simulink model "Copy_of_UAV"  (R2018b)
settings: Solver=FixedStepAuto  StartTime=0  StopTime=300  MaxStep=0.01  RelTol=1e-4  EnableMultiTasking=on
values from neighbouring files (symbols this model uses):
  actuatorCentres = 0.0    [data.sldd]
  datcom1 : value not decoded    [data.sldd]
  deflectionLimits = -10.0    [data.sldd]
  loggingSampleTime = 1.0    [data.sldd]
  sensorSampleTime = 0.02    [data.sldd]
  vehicle = 1.5    [data.sldd]
undefined symbols (not defined in the file or in its folder): aeroCoeff, DiscIntNeverNeededParam, Discrete, HDBK, MIL, Time
libraries: simulink x24, arduinolib x8, ctrlSharedLib x8, aerolibasang x5, aerolibactuator x4, aerolibadyn x3, aerolibconvert2 x2, aerolibatmos2 x2, aerolibnav x2, shared6dof x1, aerolibwind2 x1, simulink_extras x1
(part 1 of 3)
settings Model: DataDictionary=data.sldd  VariantConfigurationObject=Variants  SimulationMode=accelerator  SnapshotBufferSize=2  SnapshotInterval=1  PacingRate=10  ExtModeTrigDuration=2  Creator=Aliak  LastModifiedBy=Aliak
settings SolverCC: SolverResetMethod=Robust  MinimalZcImpactIntegration=on
settings OptimizationCC: DefaultParameterBehavior=Inlined  UseDivisionForNetSlopeComputation=on  UseFloatMulNetSlope=on  DefaultUnderspecifiedDataType=single  UseSpecifiedMinMax=on  InlineInvariantSignals=on  EnhancedBackFolding=on  BooleansAsBitfields=on  PassReuseOutputArgsAs=Individual arguments  StateBitsets=on  DataBitsets=on  ZeroExternalMemoryAtStartup=off  ZeroInternalMemoryAtStartup=off  NoFixptDivByZeroProtection=on  EfficientFloat2IntCast=on  LifeSpan=0.01  MaxStackSize=64  SimCompilerOptimization=on  OptimizeBlockOrder=speed  DifferentSizesBufferReuse=on
settings DebuggingCC: ConsistencyChecking=warning  ReadBeforeWriteMsg=DisableAll  WriteAfterWriteMsg=DisableAll  WriteAfterReadMsg=DisableAll  SolverPrmCheckMsg=warning  ParameterTunabilityLossMsg=error  UniqueDataStoreMsg=error  BusObjectLabelMismatch=error  StateNameClashWarn=warning  ForceCombineOutputUpdateInSim=on
settings HardwareCC: ProdBitPerInt=16  ProdBitPerPointer=16  ProdBitPerSizeT=16  ProdBitPerPtrDiffT=16  ProdLargestAtomicFloat=None  ProdWordSize=8  ProdLongLongMode=on  ProdHWDeviceType=Atmel->AVR
settings ModelReferenceCC: UpdateModelReferenceTargets=IfOutOfDate  EnableParallelModelReferenceBuilds=on  ModelReferenceMinAlgLoopOccurrences=on
settings SFSimCC: SimUserIncludeDirs="\"nativelibs/include\" \"nativelibs/src\" \"nativelibs/build\""  SFSimEcho=off  MATLABDynamicMemAlloc=off
settings RTWCC: SystemTargetFile=ert.tlc  HardwareBoard=Arduino Uno  TemplateMakefile=ert_default_tmf  GenerateReport=on  RTWUseSimCustomCode=on  CustomInclude="\"nativelibs/include\" \"nativelibs/src\" \"nativelibs/build\""  Toolchain=Arduino AVR  BuildConfiguration=Faster Runs  IncludeHyperlinkInReport=on  LaunchReport=on  PortableWordSizes=on  CreateSILPILBlock=PIL  GenerateTraceInfo=on  GenerateTraceReport=on  GenerateTraceReportSl=on  GenerateTraceReportSf=on  GenerateTraceReportEml=on  GenerateCodeMetricsReport=on
settings CodeAppCC: ForceParamTrailComments=on  IgnoreCustomStorageClasses=off  OperatorAnnotations=on  SimulinkDataObjDesc=on  SFDataObjDesc=on  CustomSymbolStrGlobalVar=rt$N$M  CustomSymbolStrType=$N$M  CustomSymbolStrFcn=$N$M$F  CustomSymbolStrMacro=$N$M  InsertBlockDesc=on
settings ERTTargetCC: TargetLangStandard=C99 (ISO)  UtilityFuncGeneration=Shared location  IncludeMdlTerminateFcn=off  CombineSignalStateStructs=on  SuppressErrorStatus=on  SupportNonFinite=off  SupportComplex=off  SupportVariableSizeSignals=on  CastingMode=Standards  ERTFilePackagingFormat=CompactWithDataFile

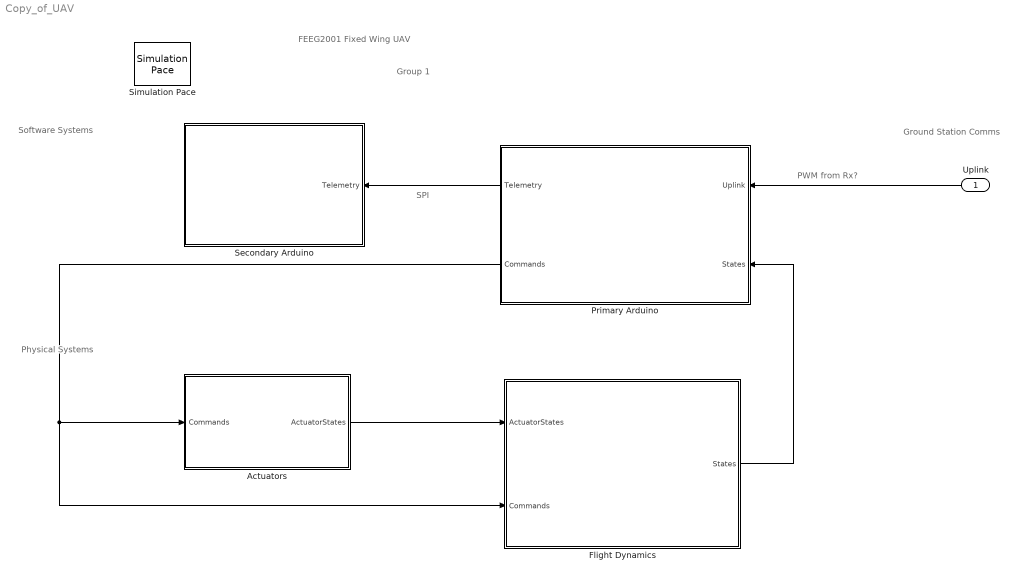
== system Copy_of_UAV ==
  note: PWM from Rx?
  note: SPI
  note: Group 1
  note: FEEG2001 Fixed Wing UAV
  note: Physical Systems
  note: Software Systems
  note: Ground Station Comms
  Uplink : Inport  OutDataTypeStr=Bus: Uplink
  Actuators : Subsystem  Variant=on
  Flight Dynamics : Subsystem
      mask Display: image('MQ-9-Reaper-armed-UAV.jpg');
  Primary Arduino : Subsystem
      mask Display: image('a000066_featured_1_.jpg');
  Secondary Arduino : Subsystem  VariantControl=Variant1
      mask Display: image('a000066_featured_1_.jpg');
  Simulation Pace : aerolibanimutils/Simulation Pace  SimulationPace=1  SleepMode=Auto  OutputPaceError=off  SampleTime=sensorSampleTime
  wires:
  Actuators/1(ActuatorStates) -> Flight Dynamics/1(ActuatorStates)
  Primary Arduino/2(Commands) -> Flight Dynamics/2(Commands), Actuators/1(Commands)
  Uplink/1 -> Primary Arduino/1(Uplink)
  Flight Dynamics/1(States) -> Primary Arduino/2(States)
  Primary Arduino/1(Telemetry) -> Secondary Arduino/1(Telemetry)

== system Copy_of_UAV/Actuators ==
  Commands : Inport
  Model Actuators : Subsystem  VariantControl=SimType == 0
  Real Actuators : Subsystem  VariantControl=SimType == 1
  ActuatorStates : Outport

== system Copy_of_UAV/Flight Dynamics ==
  ActuatorStates : Inport
  Commands : Inport  Port=2  OutDataTypeStr=Bus: Commands
  6DOF EOM : Subsystem  VariantControl=eom3DOF
  Bus Selector : BusSelector  OutputSignals=Throttle
  Coeff Model : Subsystem  Commented=on  VariantControl=AeroModel==2
  DATCOM Model : Subsystem  VariantControl=AeroModel==1
  Environment : Subsystem
  Propulsion : Subsystem
      settings: RTWSystemCode=Inline
  Sum1 : Sum  Inputs=|++  SaturateOnIntegerOverflow=on  InputSameDT=on  OutDataTypeStr=Inherit: Same as first input
  Sum2 : Sum  Inputs=|++  SaturateOnIntegerOverflow=on  InputSameDT=on  OutDataTypeStr=Inherit: Same as first input
  Visualization : Subsystem
  States : Outport
  wires:
  Commands/1 -> Bus Selector/1
  Sum2/1 -> 6DOF EOM/2(Forces)
  Propulsion/1(F) -> Sum2/2
  Propulsion/2(M) -> Sum1/2
  Sum1/1 -> 6DOF EOM/3(Moments)
  Bus Selector/1 -> Propulsion/1(cmd)  "<Throttle>"
  ActuatorStates/1 -> DATCOM Model/3(ActuatorStates)
  DATCOM Model/1(F) -> Sum2/1
  DATCOM Model/2(M) -> Sum1/1
  Environment/1(Env) -> 6DOF EOM/1(Env), DATCOM Model/1(Env)
  6DOF EOM/1(DCMbe) -> Environment/2(DCMbe)
  6DOF EOM/2(States) -> Environment/1(States), Visualization/1(States), DATCOM Model/2(States), States/1

== system Copy_of_UAV/Primary Arduino ==
  Uplink : Inport
  States : Inport  Port=2
  Communications : Subsystem
  Flight Control : Subsystem  VariantControlMode=Label  Variant=on  VariantControl=Variant1  LabelModeActiveChoice=SimType==0
  Rate Transition : RateTransition  OutPortSampleTime=loggingSampleTime
  Sensors : Subsystem  VariantControl=Variant1
  Telemetry and Errors : Subsystem  VariantControlMode=Label  Variant=on  VariantControl=Variant1  LabelModeActiveChoice=SecArd == 0
  Telemetry : Outport
  Commands : Outport  Port=2
  wires:
  Uplink/1 -> Communications/1(Uplink)
  Telemetry and Errors/1(" Telemetry") -> Telemetry/1
  States/1 -> Sensors/1(States)
  Sensors/1(Sensors) -> Rate Transition/1, Flight Control/2("Sensors ")
  Communications/1(Demands) -> Flight Control/1("Demands ")
  Flight Control/1(" Commands") -> Commands/1
  Rate Transition/1 -> Telemetry and Errors/1("Sensors ")

== system Copy_of_UAV/Secondary Arduino ==
  Telemetry : Inport
  Telemetry Logging : Subsystem  VariantControlMode=Label  Variant=on  VariantControl=Variant1  LabelModeActiveChoice=SecArd==0
  wires:
  Telemetry/1 -> Telemetry Logging/1("Telemetry ")

== system Copy_of_UAV/Actuators/Model Actuators ==
  Commands : Inport
  Bus Creator : BusCreator  Inputs=4  OutDataTypeStr=Bus: ActuatorStates
  Bus Selector : BusSelector  OutputSignals=Aileron,Elevator,Rudder,Flap
  Cast To Double{,1..3} (4 alike) : DataTypeConversion  OutDataTypeStr=double
  Linear Second-Order Actuator{,1..3} (4 alike) : aerolibactuator/Linear Second-Order Actuator  wn_fin=1  z_fin=0.3  fin_act_0=0  fin_act_vel=0
      settings: SourceProductName=Aerospace Blockset  SourceProductBaseCode=AE
  Saturation : Saturate  UpperLimit=deflectionLimits.aileron.max  LowerLimit=deflectionLimits.aileron.min
  Saturation1 : Saturate  UpperLimit=deflectionLimits.elevator.max  LowerLimit=deflectionLimits.elevator.min
  Saturation2 : Saturate  UpperLimit=deflectionLimits.rudder.max  LowerLimit=deflectionLimits.rudder.min
  Saturation3 : Saturate  UpperLimit=deflectionLimits.flap.max  LowerLimit=deflectionLimits.flap.min
  ActuatorStates : Outport
  wires:
  Bus Selector/3 -> Cast To Double2/1  "<Rudder>"
  Bus Selector/4 -> Cast To Double3/1  "<Flap>"
  Bus Selector/1 -> Cast To Double/1  "<Aileron>"
  Bus Selector/2 -> Cast To Double1/1  "<Elevator>"
  Saturation/1 -> Linear Second-Order Actuator/1
  Saturation1/1 -> Linear Second-Order Actuator1/1
  Saturation2/1 -> Linear Second-Order Actuator2/1
  Saturation3/1 -> Linear Second-Order Actuator3/1
  Linear Second-Order Actuator1/1 -> Bus Creator/2  "Elevator"
  Linear Second-Order Actuator/1 -> Bus Creator/1  "Aileron"
  Linear Second-Order Actuator2/1 -> Bus Creator/3  "Rudder"
  Linear Second-Order Actuator3/1 -> Bus Creator/4  "Flap"
  Bus Creator/1 -> ActuatorStates/1
  Commands/1 -> Bus Selector/1
  Cast To Double/1 -> Saturation/1
  Cast To Double1/1 -> Saturation1/1
  Cast To Double2/1 -> Saturation2/1
  Cast To Double3/1 -> Saturation3/1

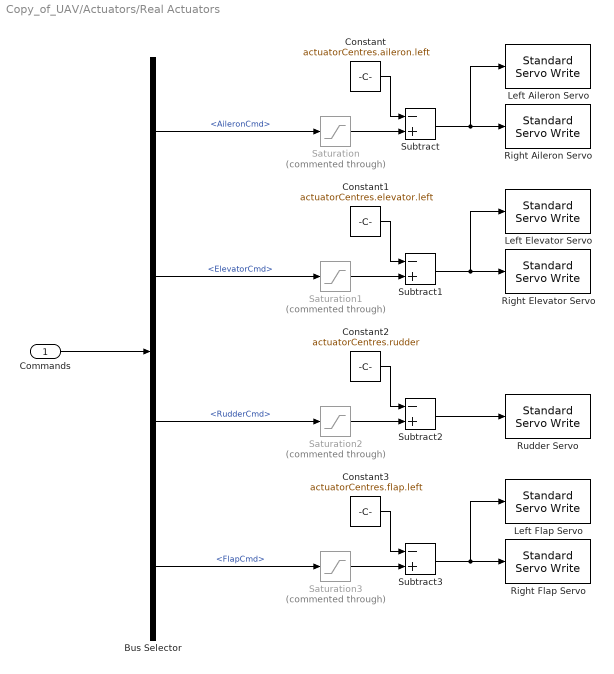
== system Copy_of_UAV/Actuators/Real Actuators ==
  Commands : Inport
  Bus Selector : BusSelector  OutputSignals=AileronCmd,ElevatorCmd,RudderCmd,FlapCmd
  Constant : Constant  Value=actuatorCentres.aileron.left
  Constant1 : Constant  Value=actuatorCentres.elevator.left
  Constant2 : Constant  Value=actuatorCentres.rudder
  Constant3 : Constant  Value=actuatorCentres.flap.left
  Left Aileron Servo : arduinolib/Standard Servo Write  pinNumber=servoPins.aileron.left  ServoIndex=0  blockPlatform=ARDUINO
      settings: SourceProductName=Simulink Support Package for Arduino Hardware
  Left Elevator Servo : arduinolib/Standard Servo Write  pinNumber=servoPins.elevator.left  ServoIndex=0  blockPlatform=ARDUINO
      settings: SourceProductName=Simulink Support Package for Arduino Hardware
  Left Flap Servo : arduinolib/Standard Servo Write  pinNumber=servoPins.flap.left  ServoIndex=0  blockPlatform=ARDUINO
      settings: SourceProductName=Simulink Support Package for Arduino Hardware
  Right Aileron Servo : arduinolib/Standard Servo Write  pinNumber=servoPins.aileron.right  ServoIndex=0  blockPlatform=ARDUINO
      settings: SourceProductName=Simulink Support Package for Arduino Hardware
  Right Elevator Servo : arduinolib/Standard Servo Write  pinNumber=servoPins.elevator.right  ServoIndex=0  blockPlatform=ARDUINO
      settings: SourceProductName=Simulink Support Package for Arduino Hardware
  Right Flap Servo : arduinolib/Standard Servo Write  pinNumber=servoPins.flap.right  ServoIndex=0  blockPlatform=ARDUINO
      settings: SourceProductName=Simulink Support Package for Arduino Hardware
  Rudder Servo : arduinolib/Standard Servo Write  pinNumber=servoPins.rudder  ServoIndex=0  blockPlatform=ARDUINO
      settings: SourceProductName=Simulink Support Package for Arduino Hardware
  Saturation : Saturate  Commented=through  UpperLimit=deflectionLimits.aileron.max  LowerLimit=deflectionLimits.aileron.min
  Saturation1 : Saturate  Commented=through  UpperLimit=deflectionLimits.elevator.max  LowerLimit=deflectionLimits.elevator.min
  Saturation2 : Saturate  Commented=through  UpperLimit=deflectionLimits.rudder.max  LowerLimit=deflectionLimits.rudder.min
  Saturation3 : Saturate  Commented=through  UpperLimit=deflectionLimits.flap.max  LowerLimit=deflectionLimits.flap.min
  Subtract{,1..3} (4 alike) : Sum  Inputs=-+
  wires:
  Saturation/1 -> Subtract/2
  Bus Selector/3 -> Saturation2/1  "<RudderCmd>"
  Commands/1 -> Bus Selector/1
  Bus Selector/4 -> Saturation3/1  "<FlapCmd>"
  Subtract3/1 -> Right Flap Servo/1, Left Flap Servo/1
  Bus Selector/1 -> Saturation/1  "<AileronCmd>"
  Constant2/1 -> Subtract2/1
  Subtract2/1 -> Rudder Servo/1
  Saturation3/1 -> Subtract3/2
  Saturation2/1 -> Subtract2/2
  Saturation1/1 -> Subtract1/2
  Bus Selector/2 -> Saturation1/1  "<ElevatorCmd>"
  Subtract/1 -> Right Aileron Servo/1, Left Aileron Servo/1
  Subtract1/1 -> Right Elevator Servo/1, Left Elevator Servo/1
  Constant/1 -> Subtract/1
  Constant1/1 -> Subtract1/1
  Constant3/1 -> Subtract3/1

== system Copy_of_UAV/Flight Dynamics/6DOF EOM ==
  Bus Element In : Inport  PortName=Env  Element=g
  Forces : Inport  Port=2
  Moments : Inport  Port=3
  6DOF (Euler Angles) : shared6dof/6DOF (Euler Angles)  units=Metric (MKS)  mtype=Fixed  rep=Euler Angles  xme_0=initConditions.x0  Vm_0=initConditions.v0  eul_0=initConditions.euler0  pm_0=initConditions.w0  mass_0=vehicle.mass  mass_e=0.5  mass_f=2.0  inertia=vehicle.inertia  inertia_e=eye(3)  inertia_f=2*eye(3)  k_quat=1.0  vre_flag=on  abi_flag=on  aMode=0  xme_statename=''  Vm_statename=''  eul_statename=''  quat_statename=''  pm_statename=''  mass_statename=''
      settings: SourceProductBaseCode=AE
  Gain : Gain  Gain=vehicle.mass
  Product : Product  Multiplication=Matrix(*)
  Sum2 : Sum  Inputs=++|  SaturateOnIntegerOverflow=on  InputSameDT=on  OutDataTypeStr=Inherit: Same as first input
  Terminator1 : Terminator
  Terminator2 : Terminator
  DCMbe : Outport
  Bus Element Out : Outport  Port=2  PortName=States  Element=phi_theta_psi
  Bus Element Out1 : Outport  Port=2  PortName=States  Element=pqr
  Bus Element Out2 : Outport  Port=2  PortName=States  Element=omega_dot
  Bus Element Out15 : Outport  Port=2  PortName=States  Element=X_e
  Bus Element Out16 : Outport  Port=2  PortName=States  Element=V_b
  Bus Element Out17 : Outport  Port=2  PortName=States  Element=A_be
  wires:
  6DOF (Euler Angles)/4 -> DCMbe/1, Product/1
  6DOF (Euler Angles)/1 -> Terminator2/1
  Bus Element In/1 -> Gain/1
  6DOF (Euler Angles)/9 -> Bus Element Out17/1
  6DOF (Euler Angles)/7 -> Bus Element Out2/1
  6DOF (Euler Angles)/6 -> Bus Element Out1/1
  6DOF (Euler Angles)/5 -> Bus Element Out16/1
  6DOF (Euler Angles)/3 -> Bus Element Out/1
  6DOF (Euler Angles)/2 -> Bus Element Out15/1
  Gain/1 -> Product/2
  Sum2/1 -> 6DOF (Euler Angles)/1
  Product/1 -> Sum2/1
  6DOF (Euler Angles)/8 -> Terminator1/1
  Moments/1 -> 6DOF (Euler Angles)/2
  Forces/1 -> Sum2/2

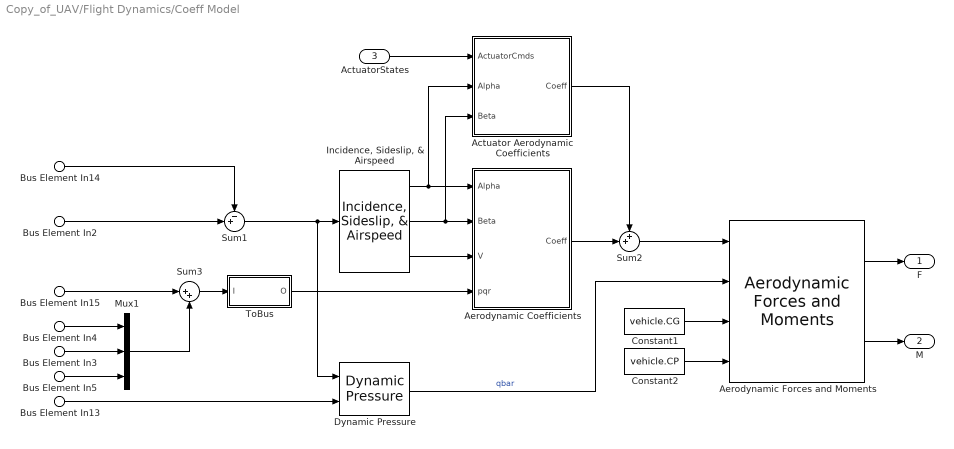
== system Copy_of_UAV/Flight Dynamics/Coeff Model ==
  Bus Element In13 : Inport  PortName=Env  Element=AirDensity
  Bus Element In14 : Inport  PortName=Env  Element=WindVelocity
  Bus Element In15 : Inport  PortName=Env  Element=WindAngularRates
  Bus Element In3 : Inport  Port=2  PortName=States  Element=q
  Bus Element In4 : Inport  Port=2  PortName=States  Element=p
  Bus Element In5 : Inport  Port=2  PortName=States  Element=r
  Bus Element In2 : Inport  Port=2  PortName=States  Element=V_b
  ActuatorStates : Inport  Port=3  OutDataTypeStr=Bus: ActuatorStates
  Actuator Aerodynamic Coefficients : Subsystem
  Aerodynamic Coefficients : Subsystem
  Aerodynamic Forces and Moments : aerolibadyn/Aerodynamic Forces and Moments   inputAxes=Body  outputForceAxes=Body  outputMomentAxes=Body  S=vehicle.wingarea  b=vehicle.wingspan  cbar=vehicle.aclength
      settings: SourceProductName=Aerospace Blockset
  Constant1 : Constant  Value=vehicle.CG
  Constant2 : Constant  Value=vehicle.CP
  Dynamic Pressure : aerolibasang/Dynamic Pressure
  "Incidence, Sideslip, & Airspeed" : aerolibasang/Incidence, Sideslip, & Airspeed
      settings: SourceProductName=Aerospace Blockset
  Mux1 : Mux  Inputs=3
  Sum1 : Sum  Inputs=-+|  SaturateOnIntegerOverflow=on  InputSameDT=on  OutDataTypeStr=Inherit: Same as first input
  Sum2 : Sum  Inputs=++|
  Sum3 : Sum  Inputs=|++  SaturateOnIntegerOverflow=on  InputSameDT=on  OutDataTypeStr=Inherit: Same as first input
  ToBus : Subsystem
  F : Outport  Unit=N
  M : Outport  Port=2  Unit=N*m
  wires:
  ActuatorStates/1 -> Actuator Aerodynamic Coefficients/1(ActuatorCmds)
  Bus Element In14/1 -> Sum1/1
  Bus Element In2/1 -> Sum1/2
  Mux1/1 -> Sum3/2
  Bus Element In15/1 -> Sum3/1
  Bus Element In5/1 -> Mux1/3
  Bus Element In3/1 -> Mux1/2
  Bus Element In4/1 -> Mux1/1
  Actuator Aerodynamic Coefficients/1(Coeff) -> Sum2/1
  Aerodynamic Coefficients/1(Coeff) -> Sum2/2
  ToBus/1(O) -> Aerodynamic Coefficients/4(pqr)
  Sum1/1 -> Dynamic Pressure/1, "Incidence, Sideslip, & Airspeed"/1
  Dynamic Pressure/1 -> Aerodynamic Forces and Moments/2  "qbar"
  Sum3/1 -> ToBus/1(I)
  Bus Element In13/1 -> Dynamic Pressure/2
  "Incidence, Sideslip, & Airspeed"/3 -> Aerodynamic Coefficients/3(V)
  "Incidence, Sideslip, & Airspeed"/2 -> Aerodynamic Coefficients/2(Beta), Actuator Aerodynamic Coefficients/3(Beta)
  Aerodynamic Forces and Moments/2 -> M/1
  Aerodynamic Forces and Moments/1 -> F/1
  Constant2/1 -> Aerodynamic Forces and Moments/4
  Constant1/1 -> Aerodynamic Forces and Moments/3
  Sum2/1 -> Aerodynamic Forces and Moments/1
  "Incidence, Sideslip, & Airspeed"/1 -> Actuator Aerodynamic Coefficients/2(Alpha), Aerodynamic Coefficients/1(Alpha)

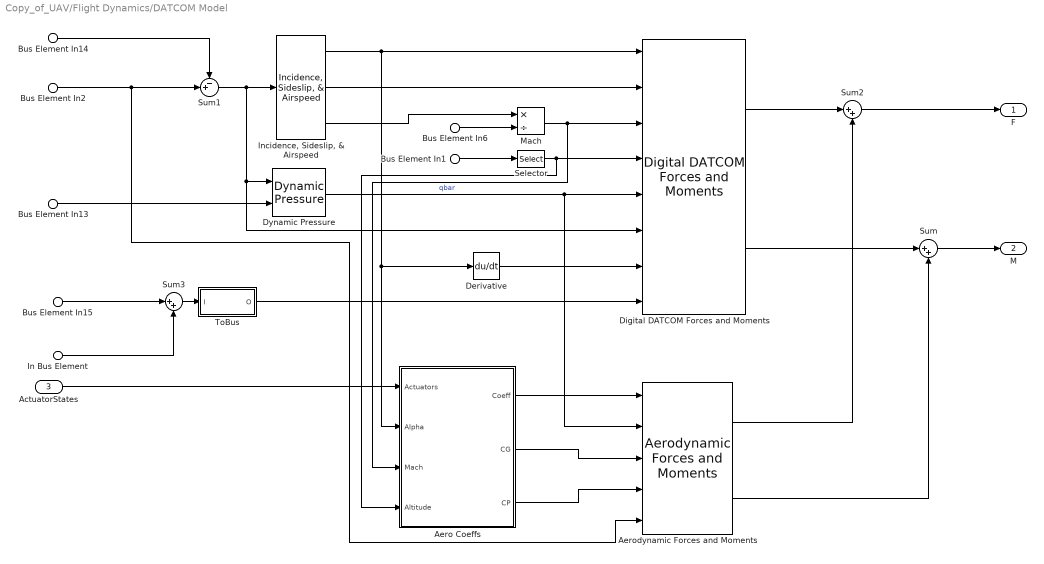
== system Copy_of_UAV/Flight Dynamics/DATCOM Model ==
  Bus Element In13 : Inport  PortName=Env  Element=AirDensity
  Bus Element In14 : Inport  PortName=Env  Element=WindVelocity
  Bus Element In15 : Inport  PortName=Env  Element=WindAngularRates
  Bus Element In6 : Inport  PortName=Env  Element=a
  Bus Element In2 : Inport  Port=2  PortName=States  Element=V_b
  Bus Element In1 : Inport  Port=2  PortName=States  Element=X_e
  In Bus Element : Inport  Port=2  PortName=States  Element=pqr
  ActuatorStates : Inport  Port=3  OutDataTypeStr=Bus: ActuatorStates
  Aero Coeffs : Subsystem
  "Aerodynamic Forces and Moments " : aerolibadyn/Aerodynamic Forces and Moments   inputAxes=Stability  outputForceAxes=Body  outputMomentAxes=Body  S=vehicle.wingarea  b=vehicle.wingspan  cbar=vehicle.cbar
      settings: SourceProductName=Aerospace Blockset
  Derivative : Derivative
  Digital DATCOM Forces and Moments : aerolibadyn/Digital DATCOM Forces and Moments  units=Metric (MKS)  dcase=datcom1{3}  fmode=Body  buildno=0  imethod=Linear  emethod=Linear  rmethod=Linear Extrapolation  action=Warning
      settings: SourceProductName=Aerospace Blockset  SourceProductBaseCode=AE
  Dynamic Pressure : aerolibasang/Dynamic Pressure
  "Incidence, Sideslip, & Airspeed" : aerolibasang/Incidence, Sideslip, & Airspeed
      settings: SourceProductName=Aerospace Blockset
  Mach : Product  Inputs=*/
  Selector : Selector  IndexMode=Zero-based  InputPortWidth=3  IndexOptions=Index vector (dialog)  Indices=[2]  OutputSizes=1
  Sum : Sum  Inputs=|++
  Sum1 : Sum  Inputs=-+|  SaturateOnIntegerOverflow=on  InputSameDT=on  OutDataTypeStr=Inherit: Same as first input
  Sum2 : Sum  Inputs=|++
  Sum3 : Sum  Inputs=|++  SaturateOnIntegerOverflow=on  InputSameDT=on  OutDataTypeStr=Inherit: Same as first input
  ToBus : Subsystem
  F : Outport  Unit=N
  M : Outport  Port=2  Unit=N*m
  wires:
  Bus Element In14/1 -> Sum1/1
  Bus Element In2/1 -> "Aerodynamic Forces and Moments "/5, Sum1/2
  In Bus Element/1 -> Sum3/2
  Bus Element In15/1 -> Sum3/1
  Sum1/1 -> "Incidence, Sideslip, & Airspeed"/1, Digital DATCOM Forces and Moments/6, Dynamic Pressure/1
  Sum3/1 -> ToBus/1(I)
  Bus Element In13/1 -> Dynamic Pressure/2
  "Incidence, Sideslip, & Airspeed"/3 -> Mach/1
  Digital DATCOM Forces and Moments/2 -> Sum/1
  Digital DATCOM Forces and Moments/1 -> Sum2/1
  Dynamic Pressure/1 -> "Aerodynamic Forces and Moments "/2, Digital DATCOM Forces and Moments/5  "qbar"
  Bus Element In1/1 -> Selector/1
  Selector/1 -> Aero Coeffs/4(Altitude), Digital DATCOM Forces and Moments/4
  Bus Element In6/1 -> Mach/2
  ActuatorStates/1 -> Aero Coeffs/1(Actuators)
  "Incidence, Sideslip, & Airspeed"/2 -> Digital DATCOM Forces and Moments/2
  "Incidence, Sideslip, & Airspeed"/1 -> Digital DATCOM Forces and Moments/1, Derivative/1, Aero Coeffs/2(Alpha)
  Aero Coeffs/1(Coeff) -> "Aerodynamic Forces and Moments "/1
  Aero Coeffs/2(CG) -> "Aerodynamic Forces and Moments "/3
  Aero Coeffs/3(CP) -> "Aerodynamic Forces and Moments "/4
  Sum/1 -> M/1
  "Aerodynamic Forces and Moments "/2 -> Sum/2
  Sum2/1 -> F/1
  "Aerodynamic Forces and Moments "/1 -> Sum2/2
  ToBus/1(O) -> Digital DATCOM Forces and Moments/8
  Derivative/1 -> Digital DATCOM Forces and Moments/7
  Mach/1 -> Digital DATCOM Forces and Moments/3, Aero Coeffs/3(Mach)

== system Copy_of_UAV/Flight Dynamics/Environment ==
  States : Inport
  DCMbe : Inport  Port=2
  Bus Creator : BusCreator  Inputs=5
  Bus Selector : BusSelector  OutputSignals=X_e,V_b
  Dryden Wind Turbulence Model (Discrete (-q +r)) : aerolibwind2/Dryden Wind Turbulence Model  (Continuous (+q -r))  units=Metric (MKS)  spec=MIL-HDBK-1797  model=Discrete Dryden (-q +r)  W20=1  Wdeg=250  TurbProb=10^-1  L_high=533.4  Wingspan=1.8  ts=sensorSampleTime  Seed=[23341 23342 23343 23344]  T_on=off
      settings: SourceProductName=Aerospace Blockset
  Lapse Rate Model : aerolibatmos2/ISA Atmosphere Model  custom=off  g=9.80665  gamma=1.4  R=287.0531  L=0.0065  h_trop=11000  h_strat=20000  rho0=1.225  P0=101325  T0=288.15  h0=0
      settings: SourceProductName=Aerospace Blockset
  Selector : Selector  IndexMode=Zero-based  InputPortWidth=3  IndexOptions=Index vector (dialog)  Indices=[0]  OutputSizes=1
  Selector1 : Selector  IndexMode=Zero-based  InputPortWidth=3  IndexOptions=Index vector (dialog)  Indices=[0]  OutputSizes=1
  Terminator : Terminator
  Terminator1 : Terminator
  g : Constant  Value=[0 0 9.80665]
  Env : Outport
  wires:
  States/1 -> Bus Selector/1
  Bus Creator/1 -> Env/1
  Selector/1 -> Dryden Wind Turbulence Model (Discrete (-q +r))/1, Lapse Rate Model/1
  Bus Selector/1 -> Selector/1  "<X_e>"
  Lapse Rate Model/4 -> Bus Creator/2  "AirDensity"
  Lapse Rate Model/2 -> Bus Creator/1  "a"
  g/1 -> Bus Creator/3  "g"
  DCMbe/1 -> Dryden Wind Turbulence Model (Discrete (-q +r))/3
  Bus Selector/2 -> Selector1/1  "<V_b>"
  Selector1/1 -> Dryden Wind Turbulence Model (Discrete (-q +r))/2
  Dryden Wind Turbulence Model (Discrete (-q +r))/1 -> Bus Creator/4  "WindVelocity"
  Dryden Wind Turbulence Model (Discrete (-q +r))/2 -> Bus Creator/5  "WindAngularRates"
  Lapse Rate Model/1 -> Terminator/1
  Lapse Rate Model/3 -> Terminator1/1

== system Copy_of_UAV/Flight Dynamics/Propulsion ==
  cmd : Inport  OutDataTypeStr=single
  Cast To Double : DataTypeConversion  OutDataTypeStr=double
  Mux : Mux  Inputs=[1 2]
  Product : Product
  ThrustX : Lookup_n-D  NumberOfTableDimensions=1  LookupTableObject=''  BreakpointsForDimension1=(1/6)*(3+([-3:3]))  IndexSearchMethod=Linear search  BeginIndexSearchUsingPreviousIndexResult=on  Table=vehicle.thrust*(1+tanh([-3:3]))  ExtrapMethod=Clip  InternalRulePriority=Speed
  ThrustYZ : Constant  Value=[0 0]'  SampleTime=-1
  Thrust_M1 : Constant  Value=[-0.1 0 0.01]  SampleTime=-1
  Vector Concatenate : Concatenate
  F : Outport  Unit=N
  M : Outport  Port=2  Unit=N*m
  wires:
  Thrust_M1/1 -> Product/2
  ThrustX/1 -> Mux/1, Vector Concatenate/2
  ThrustYZ/1 -> Vector Concatenate/1, Mux/2
  Mux/1 -> F/1
  cmd/1 -> Cast To Double/1
  Product/1 -> M/1
  Vector Concatenate/1 -> Product/1
  Cast To Double/1 -> ThrustX/1

== system Copy_of_UAV/Flight Dynamics/Visualization ==
  Bus Element In3 : Inport  PortName=States  Element=pqr
  Bus Element In9 : Inport  PortName=States  Element=X_e
  In Bus Element : Inport  PortName=States  Element=V_b
  In Bus Element1 : Inport  PortName=States  Element=phi_theta_psi
  "Incidence, Sideslip, & Airspeed" : aerolibasang/Incidence, Sideslip, & Airspeed
      settings: SourceProductName=Aerospace Blockset
  Mux5 : Mux  Inputs=2
  State Plots : Scope  NumInputPorts=4
  Terminator : Terminator
  wires:
  Bus Element In9/1 -> State Plots/4
  In Bus Element1/1 -> State Plots/2
  Mux5/1 -> State Plots/1
  "Incidence, Sideslip, & Airspeed"/2 -> Mux5/2  "beta"
  "Incidence, Sideslip, & Airspeed"/1 -> Mux5/1  "alpha"
  In Bus Element/1 -> "Incidence, Sideslip, & Airspeed"/1
  Bus Element In3/1 -> State Plots/3
  "Incidence, Sideslip, & Airspeed"/3 -> Terminator/1

== system Copy_of_UAV/Primary Arduino/Communications ==
  Uplink : Inport  OutDataTypeStr=Bus: Uplink
  Bus Creator : BusCreator  Inputs=5  OutDataTypeStr=Bus: Demands
      settings: InheritFromInputs=off
  Bus Selector : BusSelector  OutputSignals=AutoflightRefValues,Override,ControlOverride
  Bus Selector1 : BusSelector  OutputSignals=FlightMode,HoldAltitude,HoldHeading
  Demands : Outport  OutDataTypeStr=Bus: Demands
  wires:
  Uplink/1 -> Bus Selector/1
  Bus Selector/1 -> Bus Selector1/1  "<AutoflightRefValues>"
  Bus Selector1/1 -> Bus Creator/1  "<FlightMode>"
  Bus Selector1/2 -> Bus Creator/2  "<HoldAltitude>"
  Bus Selector1/3 -> Bus Creator/3  "<HoldHeading>"
  Bus Creator/1 -> Demands/1
  Bus Selector/3 -> Bus Creator/5  "<ControlOverride>"
  Bus Selector/2 -> Bus Creator/4  "<Override>"

== system Copy_of_UAV/Primary Arduino/Flight Control ==
  "Demands " : Inport
  "Sensors " : Inport  Port=2
  Model Flight Control : Subsystem  VariantControl=SimType==0
  Real Flight Control : Subsystem  VariantControl=SimType==1
  " Commands" : Outport

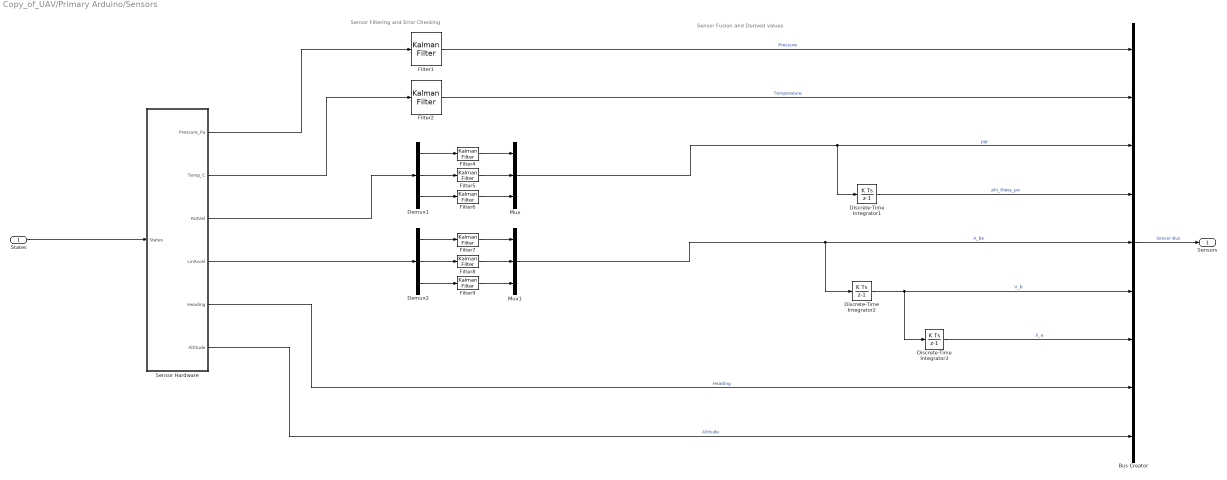
== system Copy_of_UAV/Primary Arduino/Sensors ==
  note: Sensor Fusion and Derived values
  note: Sensor Filtering and Error Checking
  States : Inport
  Bus Creator : BusCreator  Inputs=9  OutDataTypeStr=Bus: Sensors
  Demux1 : Demux  Outputs=3
  Demux2 : Demux  Outputs=3
  Discrete-Time Integrator1 : DiscreteIntegrator  SampleTime=sensorSampleTime  ICPrevOutput=DiscIntNeverNeededParam  ICPrevScaledInput=DiscIntNeverNeededParam
  Discrete-Time Integrator2 : DiscreteIntegrator  SampleTime=sensorSampleTime  ICPrevOutput=DiscIntNeverNeededParam  ICPrevScaledInput=DiscIntNeverNeededParam
  Discrete-Time Integrator3 : DiscreteIntegrator  SampleTime=sensorSampleTime  ICPrevOutput=DiscIntNeverNeededParam  ICPrevScaledInput=DiscIntNeverNeededParam
  Filter1 : ctrlSharedLib/Kalman Filter  TimeDomain=Discrete-Time  UseCurrentEstimator=on  ModelSource=Individual A, B, C, D matrices  ModelSourceVariable=ss(1,[],1,[],1)  A=0.95  B=1  C=1  D=0  NumberOfStates=1  NumberOfInputs=1  NumberOfOutputs=1  InitialEstimateSource=Dialog  X0=101325  P0=10  UseK=off  UseGH=off  NumberOfProcessNoiseInputs=1  G=1  TimeInvariantG=on  H=0  TimeInvariantH=on  Q=0.05  TimeInvariantQ=on  R=1  TimeInvariantR=on  N=0  TimeInvariantN=on  AddInputPort=off  AddEnablePort=off  OutputEstimatedY=off  OutputP=off  Ts=sensorSampleTime
      settings: SourceProductBaseCode=CT
  Filter2 : ctrlSharedLib/Kalman Filter  TimeDomain=Discrete-Time  UseCurrentEstimator=on  ModelSource=Individual A, B, C, D matrices  ModelSourceVariable=ss(1,[],1,[],1)  A=0.95  B=1  C=1  D=0  NumberOfStates=1  NumberOfInputs=1  NumberOfOutputs=1  InitialEstimateSource=Dialog  X0=15  P0=10  UseK=off  UseGH=off  NumberOfProcessNoiseInputs=1  G=1  TimeInvariantG=on  H=0  TimeInvariantH=on  Q=0.05  TimeInvariantQ=on  R=1  TimeInvariantR=on  N=0  TimeInvariantN=on  AddInputPort=off  AddEnablePort=off  OutputEstimatedY=off  OutputP=off  Ts=sensorSampleTime
      settings: SourceProductBaseCode=CT
  Filter4 : ctrlSharedLib/Kalman Filter  TimeDomain=Discrete-Time  UseCurrentEstimator=on  ModelSource=Individual A, B, C, D matrices  ModelSourceVariable=ss(0.95,[],1,[],1/95)  A=0.95  B=1  C=1  D=0  NumberOfStates=1  NumberOfInputs=1  NumberOfOutputs=1  InitialEstimateSource=Dialog  X0=0  P0=10  UseK=off  UseGH=off  NumberOfProcessNoiseInputs=1  G=1  TimeInvariantG=on  H=0  TimeInvariantH=on  Q=0.05  TimeInvariantQ=on  R=0.8  TimeInvariantR=on  N=0  TimeInvariantN=on  AddInputPort=off  AddEnablePort=off  OutputEstimatedY=off  OutputP=off  Ts=sensorSampleTime
      settings: SourceProductBaseCode=CT
  Filter5 : ctrlSharedLib/Kalman Filter  TimeDomain=Discrete-Time  UseCurrentEstimator=on  ModelSource=Individual A, B, C, D matrices  ModelSourceVariable=ss(0.95,[],1,[],1/95)  A=0.95  B=1  C=1  D=0  NumberOfStates=1  NumberOfInputs=1  NumberOfOutputs=1  InitialEstimateSource=Dialog  X0=0  P0=10  UseK=off  UseGH=off  NumberOfProcessNoiseInputs=1  G=1  TimeInvariantG=on  H=0  TimeInvariantH=on  Q=0.05  TimeInvariantQ=on  R=0.8  TimeInvariantR=on  N=0  TimeInvariantN=on  AddInputPort=off  AddEnablePort=off  OutputEstimatedY=off  OutputP=off  Ts=sensorSampleTime
      settings: SourceProductBaseCode=CT
  Filter6 : ctrlSharedLib/Kalman Filter  TimeDomain=Discrete-Time  UseCurrentEstimator=on  ModelSource=Individual A, B, C, D matrices  ModelSourceVariable=ss(0.95,[],1,[],1/95)  A=0.95  B=1  C=1  D=0  NumberOfStates=1  NumberOfInputs=1  NumberOfOutputs=1  InitialEstimateSource=Dialog  X0=0  P0=10  UseK=off  UseGH=off  NumberOfProcessNoiseInputs=1  G=1  TimeInvariantG=on  H=0  TimeInvariantH=on  Q=0.05  TimeInvariantQ=on  R=0.8  TimeInvariantR=on  N=0  TimeInvariantN=on  AddInputPort=off  AddEnablePort=off  OutputEstimatedY=off  OutputP=off  Ts=sensorSampleTime
      settings: SourceProductBaseCode=CT
  Filter7 : ctrlSharedLib/Kalman Filter  TimeDomain=Discrete-Time  UseCurrentEstimator=on  ModelSource=Individual A, B, C, D matrices  ModelSourceVariable=ss(0.95,[],1,[],1/100)  A=0.95  B=1  C=1  D=0  NumberOfStates=1  NumberOfInputs=1  NumberOfOutputs=1  InitialEstimateSource=Dialog  X0=0  P0=10  UseK=off  UseGH=off  NumberOfProcessNoiseInputs=1  G=1  TimeInvariantG=on  H=0  TimeInvariantH=on  Q=0.05  TimeInvariantQ=on  R=1  TimeInvariantR=on  N=0  TimeInvariantN=on  AddInputPort=off  AddEnablePort=off  OutputEstimatedY=off  OutputP=off  Ts=sensorSampleTime
      settings: SourceProductBaseCode=CT
  Filter8 : ctrlSharedLib/Kalman Filter  TimeDomain=Discrete-Time  UseCurrentEstimator=on  ModelSource=Individual A, B, C, D matrices  ModelSourceVariable=ss(0.95,[],1,[],1/100)  A=0.95  B=1  C=1  D=0  NumberOfStates=1  NumberOfInputs=1  NumberOfOutputs=1  InitialEstimateSource=Dialog  X0=0  P0=10  UseK=off  UseGH=off  NumberOfProcessNoiseInputs=1  G=1  TimeInvariantG=on  H=0  TimeInvariantH=on  Q=0.05  TimeInvariantQ=on  R=1  TimeInvariantR=on  N=0  TimeInvariantN=on  AddInputPort=off  AddEnablePort=off  OutputEstimatedY=off  OutputP=off  Ts=sensorSampleTime
      settings: SourceProductBaseCode=CT
  Filter9 : ctrlSharedLib/Kalman Filter  TimeDomain=Discrete-Time  UseCurrentEstimator=on  ModelSource=Individual A, B, C, D matrices  ModelSourceVariable=ss(0.95,[],1,[],1/100)  A=0.95  B=1  C=1  D=0  NumberOfStates=1  NumberOfInputs=1  NumberOfOutputs=1  InitialEstimateSource=Dialog  X0=0  P0=10  UseK=off  UseGH=off  NumberOfProcessNoiseInputs=1  G=1  TimeInvariantG=on  H=0  TimeInvariantH=on  Q=0.05  TimeInvariantQ=on  R=1  TimeInvariantR=on  N=0  TimeInvariantN=on  AddInputPort=off  AddEnablePort=off  OutputEstimatedY=off  OutputP=off  Ts=sensorSampleTime
      settings: SourceProductBaseCode=CT
  Mux : Mux  Inputs=3
  Mux1 : Mux  Inputs=3
  Sensor Hardware : Subsystem  VariantControlMode=Label  Variant=on  VariantControl=Variant1  LabelModeActiveChoice=SimType==1
  Sensors : Outport
  wires:
  Demux1/3 -> Filter6/1
  Demux1/2 -> Filter5/1
  Discrete-Time Integrator1/1 -> Bus Creator/4  "phi_theta_psi"
  Mux/1 -> Discrete-Time Integrator1/1, Bus Creator/3  "pqr"
  Demux2/1 -> Filter7/1
  Filter1/1 -> Bus Creator/1  "Pressure"
  Discrete-Time Integrator2/1 -> Discrete-Time Integrator3/1, Bus Creator/6  "V_b"
  Filter4/1 -> Mux/1
  Demux1/1 -> Filter4/1
  Filter9/1 -> Mux1/3
  Demux2/3 -> Filter9/1
  Demux2/2 -> Filter8/1
  Filter6/1 -> Mux/3
  Filter8/1 -> Mux1/2
  Filter5/1 -> Mux/2
  Filter2/1 -> Bus Creator/2  "Temperature"
  Discrete-Time Integrator3/1 -> Bus Creator/7  "X_e"
  Filter7/1 -> Mux1/1
  Mux1/1 -> Discrete-Time Integrator2/1, Bus Creator/5  "A_be"
  Bus Creator/1 -> Sensors/1  "Sensor Bus"
  States/1 -> Sensor Hardware/1("States ")
  Sensor Hardware/1(" Pressure_Pa") -> Filter1/1
  Sensor Hardware/2(" Temp_C") -> Filter2/1
  Sensor Hardware/3(" RotVel") -> Demux1/1
  Sensor Hardware/4(" LinAccel") -> Demux2/1
  Sensor Hardware/5(" Heading") -> Bus Creator/8  "Heading"
  Sensor Hardware/6(" Altitude") -> Bus Creator/9  "Altitude"

== system Copy_of_UAV/Primary Arduino/Telemetry and Errors ==
  "Sensors " : Inport  SampleTime=loggingSampleTime
  SPI Logging to Secondary : Subsystem  VariantControl=SecArd == 1
  Simulink Logging : Subsystem  VariantControl=SecArd == 0
  " Telemetry" : Outport

== system Copy_of_UAV/Secondary Arduino/Telemetry Logging ==
  "Telemetry " : Inport
  SD Logging : Subsystem  VariantControl=SecArd==1
  Simulink Logging : Subsystem  VariantControl=SecArd==0

== system Copy_of_UAV/Flight Dynamics/Coeff Model/Actuator Aerodynamic Coefficients ==
  Bus Element In13 : Inport  PortName=ActuatorCmds  Element=Elevator
  Bus Element In1 : Inport  PortName=ActuatorCmds  Element=Aileron
  Bus Element In2 : Inport  PortName=ActuatorCmds  Element=Rudder
  Alpha : Inport  Port=2
  Beta : Inport  Port=3
  Aileron : Subsystem
  Constant : Constant  Value=0
  Elevator : Subsystem
  Flap : Subsystem
  Rudder : Subsystem
  Sum : Sum  Inputs=4  SaturateOnIntegerOverflow=on  InputSameDT=on  OutDataTypeStr=Inherit: Same as first input
  Coeff : Outport  InitialOutput=0
  wires:
  Constant/1 -> Flap/1(Actuator)
  Bus Element In2/1 -> Rudder/1(Actuator)
  Bus Element In1/1 -> Aileron/1(Actuator)
  Bus Element In13/1 -> Elevator/1(Actuator)
  Beta/1 -> Elevator/2(Beta)
  Flap/1(delCoeff) -> Sum/4
  Alpha/1 -> Flap/2(Alpha), Rudder/2(Alpha), Aileron/2(Alpha)
  Rudder/1(delCoeff) -> Sum/3
  Aileron/1(delCoeff) -> Sum/2
  Elevator/1(delCoeff) -> Sum/1
  Sum/1 -> Coeff/1

== system Copy_of_UAV/Flight Dynamics/Coeff Model/Aerodynamic Coefficients ==
  Alpha : Inport
  Beta : Inport  Port=2
  V : Inport  Port=3
  pqr : Inport  Port=4  Unit=m/s
  Body Rate Damping : Subsystem
  Datum Coefficients : Subsystem
  Sum : Sum  Inputs=|++
  Coeff : Outport
  wires:
  pqr/1 -> Body Rate Damping/2(pqr)
  Sum/1 -> Coeff/1
  V/1 -> Body Rate Damping/1(V)
  Body Rate Damping/1(Coeff) -> Sum/2
  Datum Coefficients/1(Coeff) -> Sum/1
  Beta/1 -> Datum Coefficients/2(Beta)
  Alpha/1 -> Datum Coefficients/1(Alpha)

== system Copy_of_UAV/Flight Dynamics/Coeff Model/ToBus ==
  I : Inport
  Bus Creator3 : BusCreator  Inputs=3
  Demux : Demux  Outputs=3
  O : Outport
  wires:
  I/1 -> Demux/1
  Demux/2 -> Bus Creator3/2  "q_wind"
  Bus Creator3/1 -> O/1
  Demux/3 -> Bus Creator3/3  "r_wind"
  Demux/1 -> Bus Creator3/1  "p_wind"

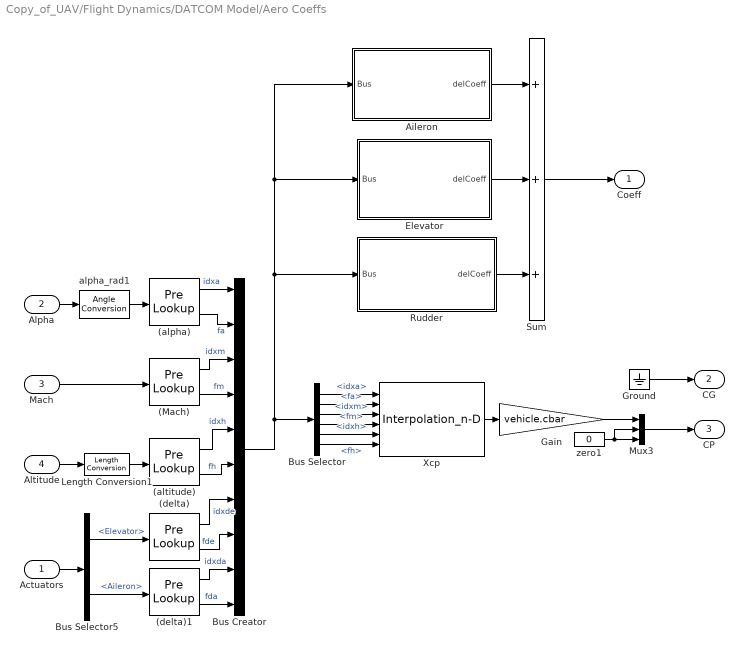
== system Copy_of_UAV/Flight Dynamics/DATCOM Model/Aero Coeffs ==
  Actuators : Inport
  Alpha : Inport  Port=2
  Mach : Inport  Port=3
  Altitude : Inport  Port=4
  (Mach) : PreLookup  BreakpointsData=datcom1{3}.mach  BeginIndexSearchUsingPreviousIndexResult=on  ExtrapMethod=Linear  IndexDataTypeStr=int32  FractionDataTypeStr=double
  (alpha) : PreLookup  BreakpointsData=datcom1{3}.alpha  BeginIndexSearchUsingPreviousIndexResult=on  ExtrapMethod=Linear  IndexDataTypeStr=int32  FractionDataTypeStr=double
  (altitude) : PreLookup  BreakpointsData=datcom1{3}.alt  BeginIndexSearchUsingPreviousIndexResult=on  ExtrapMethod=Linear  IndexDataTypeStr=int32  FractionDataTypeStr=double
  (delta) : PreLookup  BreakpointsData=datcom1{3}.delta  BeginIndexSearchUsingPreviousIndexResult=on  ExtrapMethod=Linear  IndexDataTypeStr=int32  FractionDataTypeStr=double
  (delta)1 : PreLookup  BreakpointsData=datcom1{2}.deltal  BeginIndexSearchUsingPreviousIndexResult=on  ExtrapMethod=Linear  IndexDataTypeStr=int32  FractionDataTypeStr=double
  Aileron : Subsystem
  Bus Creator : BusCreator  Inputs=10
  Bus Selector : BusSelector  OutputSignals=idxa,fa,idxm,fm,idxh,fh
  Bus Selector5 : BusSelector  OutputSignals=Elevator,Aileron
  Elevator : Subsystem
  Gain : Gain  Gain=vehicle.cbar
  Ground : Ground
  Length Conversion1 : aerolibconvert2/Length Conversion  IU=m  OU=ft
  Mux3 : Mux  Inputs=3
  Rudder : Subsystem
  Sum : Sum  Inputs=3  SaturateOnIntegerOverflow=on  InputSameDT=on  OutDataTypeStr=Inherit: Same as first input
  Xcp : Interpolation_n-D  NumberOfTableDimensions=3  Table="permute(datcom1{1}.xcp,[1  2  3])"  OutDataTypeStr=double
      settings: InputPortMap=u0,u1,u2,u3,u4,u5
  alpha_rad1 : aerolibconvert2/Angle Conversion  IU=rad  OU=deg
  zero1 : Constant  Value=0
  Coeff : Outport
  CG : Outport  Port=2  PortDimensions=3
  CP : Outport  Port=3  PortDimensions=3
  wires:
  Aileron/1(delCoeff) -> Sum/1
  Sum/1 -> Coeff/1
  (alpha)/1 -> Bus Creator/1  "idxa"
  Gain/1 -> Mux3/1
  (delta)/2 -> Bus Creator/8  "fde"
  (alpha)/2 -> Bus Creator/2  "fa"
  Bus Selector/5 -> Xcp/5  "<idxh>"
  alpha_rad1/1 -> (alpha)/1
  Elevator/1(delCoeff) -> Sum/2
  Alpha/1 -> alpha_rad1/1
  Bus Selector/4 -> Xcp/4  "<fm>"
  Bus Selector/3 -> Xcp/3  "<idxm>"
  Mach/1 -> (Mach)/1
  (delta)/1 -> Bus Creator/7  "idxde"
  zero1/1 -> Mux3/2, Mux3/3
  Length Conversion1/1 -> (altitude)/1
  Bus Selector/1 -> Xcp/1  "<idxa>"
  Bus Creator/1 -> Bus Selector/1, Aileron/1(Bus), Elevator/1(Bus), Rudder/1(Bus)
  Bus Selector/2 -> Xcp/2  "<fa>"
  Actuators/1 -> Bus Selector5/1
  (Mach)/1 -> Bus Creator/3  "idxm"
  (Mach)/2 -> Bus Creator/4  "fm"
  Rudder/1(delCoeff) -> Sum/3
  Altitude/1 -> Length Conversion1/1
  Ground/1 -> CG/1
  Mux3/1 -> CP/1
  (altitude)/2 -> Bus Creator/6  "fh"
  (altitude)/1 -> Bus Creator/5  "idxh"
  Xcp/1 -> Gain/1
  Bus Selector5/1 -> (delta)/1  "<Elevator>"
  Bus Selector/6 -> Xcp/6  "<fh>"
  Bus Selector5/2 -> (delta)1/1  "<Aileron>"
  (delta)1/1 -> Bus Creator/9  "idxda"
  (delta)1/2 -> Bus Creator/10  "fda"

== system Copy_of_UAV/Flight Dynamics/DATCOM Model/ToBus ==
  I : Inport
  Bus Creator3 : BusCreator  Inputs=3
  Demux : Demux  Outputs=3
  O : Outport
  wires:
  I/1 -> Demux/1
  Demux/2 -> Bus Creator3/2  "q_wind"
  Bus Creator3/1 -> O/1
  Demux/3 -> Bus Creator3/3  "r_wind"
  Demux/1 -> Bus Creator3/1  "p_wind"

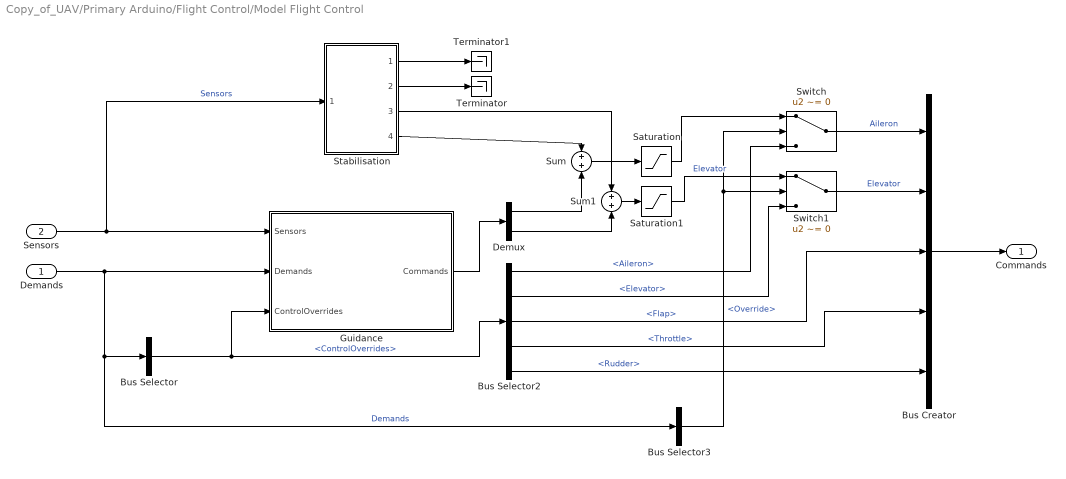
== system Copy_of_UAV/Primary Arduino/Flight Control/Model Flight Control ==
  Demands : Inport  OutDataTypeStr=Bus: Demands
  Sensors : Inport  Port=2  OutDataTypeStr=Bus: Sensors
  Bus Creator : BusCreator  Inputs=5  OutDataTypeStr=Bus: Commands
      settings: InheritFromInputs=off
  Bus Selector : BusSelector  OutputSignals=ControlOverrides
  Bus Selector2 : BusSelector  OutputSignals=Aileron,Elevator,Flap,Throttle,Rudder
  Bus Selector3 : BusSelector  OutputSignals=Override
  Demux : Demux  Outputs=2
  Guidance : Stateflow chart  TreatAsAtomicUnit=on
  Saturation : Saturate  UpperLimit=deflectionLimits.aileron.max  LowerLimit=deflectionLimits.aileron.min
  Saturation1 : Saturate  UpperLimit=deflectionLimits.elevator.max  LowerLimit=deflectionLimits.elevator.min
  Stabilisation : Subsystem
  Sum : Sum
  Sum1 : Sum
  Switch : Switch  Criteria=u2 ~= 0
  Switch1 : Switch  Criteria=u2 ~= 0
  Terminator : Terminator
  Terminator1 : Terminator
  Commands : Outport
  wires:
  Bus Creator/1 -> Commands/1
  Sum/1 -> Saturation/1
  Sum1/1 -> Saturation1/1
  Saturation/1 -> Switch/1
  Switch1/1 -> Bus Creator/2  "Elevator"
  Guidance/1(Commands) -> Demux/1
  Demux/1 -> Sum/2
  Sensors/1 -> Stabilisation/1(Sensors), Guidance/1(Sensors)  "Sensors"
  Demands/1 -> Bus Selector3/1, Bus Selector/1, Guidance/2(Demands)  "Demands"
  Bus Selector/1 -> Guidance/3(ControlOverrides), Bus Selector2/1  "<ControlOverrides>"
  Demux/2 -> Sum1/2
  Stabilisation/4(Roll Stab) -> Sum/1
  Stabilisation/3(Pitch Stab) -> Sum1/1
  Stabilisation/2(Yaw Stab) -> Terminator/1
  Bus Selector2/4 -> Bus Creator/4  "<Throttle>"
  Bus Selector2/5 -> Bus Creator/5  "<Rudder>"
  Stabilisation/1(Stall Stab) -> Terminator1/1
  Bus Selector2/3 -> Bus Creator/3  "<Flap>"
  Switch/1 -> Bus Creator/1  "Aileron"
  Bus Selector2/1 -> Switch/3  "<Aileron>"
  Bus Selector2/2 -> Switch1/3  "<Elevator>"
  Saturation1/1 -> Switch1/1  "Elevator"
  Bus Selector3/1 -> Switch/2, Switch1/2  "<Override>"

== system Copy_of_UAV/Primary Arduino/Flight Control/Real Flight Control ==
  note: These controls are overriden in hardware and untouchable by the flight computer as per spec
  Demands : Inport  OutDataTypeStr=Bus: Demands
  Sensors : Inport  Port=2  OutDataTypeStr=Bus: Sensors
  Bus Creator : BusCreator  Inputs=5  OutDataTypeStr=Bus: Commands
      settings: InheritFromInputs=off
  Constant : Constant  Value=0
  Constant1 : Constant  Value=0
  Constant2 : Constant  Value=0
  Demux : Demux  Outputs=2
  Guidance : Stateflow chart  TreatAsAtomicUnit=on
  Saturation : Saturate  UpperLimit=deflectionLimits.aileron.max  LowerLimit=deflectionLimits.aileron.min
  Saturation1 : Saturate  UpperLimit=deflectionLimits.elevator.max  LowerLimit=deflectionLimits.elevator.min
  Stabilisation : Subsystem
  Sum : Sum
  Sum1 : Sum  Inputs=+++
  Terminator : Terminator
  Commands : Outport
  wires:
  Bus Creator/1 -> Commands/1
  Sum/1 -> Saturation/1
  Sum1/1 -> Saturation1/1
  Guidance/1(Commands) -> Demux/1
  Demux/1 -> Sum/2
  Sensors/1 -> Stabilisation/1(Sensors), Guidance/1(Sensors)  "Sensors"
  Demands/1 -> Guidance/2(Demands)  "Demands"
  Demux/2 -> Sum1/3
  Stabilisation/2(Roll Stab) -> Sum/1
  Stabilisation/3(Pitch Stab) -> Sum1/1
  Stabilisation/1(Yaw Stab) -> Terminator/1
  Stabilisation/4(Stall Stab) -> Sum1/2
  Saturation/1 -> Bus Creator/1  "Aileron"
  Saturation1/1 -> Bus Creator/2  "Elevator"
  Constant/1 -> Bus Creator/3  "Flap"
  Constant1/1 -> Bus Creator/4  "Throttle"
  Constant2/1 -> Bus Creator/5  "Rudder"

== system Copy_of_UAV/Primary Arduino/Sensors/Sensor Hardware ==
  "States " : Inport
  Model Sensors : Subsystem  VariantControl=SimType==0
  Real Sensors : Subsystem  VariantControl=SimType==1
  " Pressure_Pa" : Outport
  " Temp_C" : Outport  Port=2
  " RotVel" : Outport  Port=3
  " LinAccel" : Outport  Port=4
  " Heading" : Outport  Port=5
  " Altitude" : Outport  Port=6

== system Copy_of_UAV/Primary Arduino/Telemetry and Errors/SPI Logging to Secondary ==
  note: Nothing meaningful is sent back
  "Sensors " : Inport
  Bus Selector : BusSelector  OutputSignals=X_e,phi_theta_psi,pqr,V_b,Heading
  Demux{,1..3} (4 alike) : Demux  Outputs=3
  SPI WriteRead : arduinolib/SPI WriteRead  slaveSelectPin_=10  blockPlatform=arduino
      settings: SourceProductName=Simulink Support Package for Arduino Hardware  SourceProductBaseCode=ARDUINO
  Terminator : Terminator
  Vector Concatenate : Concatenate  NumInputs=13
  wires:
  SPI WriteRead/1 -> Terminator/1
  "Sensors "/1 -> Bus Selector/1
  Bus Selector/1 -> Demux/1  "<X_e>"
  Bus Selector/2 -> Demux1/1  "<phi_theta_psi>"
  Bus Selector/3 -> Demux2/1  "<pqr>"
  Bus Selector/4 -> Demux3/1  "<V_b>"
  Bus Selector/5 -> Vector Concatenate/13  "<Heading>"
  Demux/1 -> Vector Concatenate/1
  Demux/2 -> Vector Concatenate/2
  Demux/3 -> Vector Concatenate/3
  Demux1/1 -> Vector Concatenate/4
  Demux1/2 -> Vector Concatenate/5
  Demux1/3 -> Vector Concatenate/6
  Demux2/1 -> Vector Concatenate/7
  Demux2/2 -> Vector Concatenate/8
  Demux2/3 -> Vector Concatenate/9
  Demux3/1 -> Vector Concatenate/10
  Demux3/2 -> Vector Concatenate/11
  Demux3/3 -> Vector Concatenate/12
  Vector Concatenate/1 -> SPI WriteRead/1

== system Copy_of_UAV/Primary Arduino/Telemetry and Errors/Simulink Logging ==
  "Sensors " : Inport  OutDataTypeStr=Bus: Sensors
  Telemetry : Outport
  wires:
  "Sensors "/1 -> Telemetry/1

== system Copy_of_UAV/Secondary Arduino/Telemetry Logging/SD Logging ==

== system Copy_of_UAV/Secondary Arduino/Telemetry Logging/Simulink Logging ==
  Telemetry : Inport
  Altitude : Scope
  Body Angles : Scope  NumInputPorts=3
  Body Velocities : Scope  NumInputPorts=3
  Bus Selector : BusSelector  OutputSignals=phi_theta_psi,V_b,Altitude,Heading
  Demux : Demux  Outputs=3
  Demux1 : Demux  Outputs=3
  Heading : Scope
  wires:
  Demux1/3 -> Body Velocities/3  "Z Vel"
  Demux1/2 -> Body Velocities/2  "Y Vel"
  Bus Selector/3 -> Altitude/1  "<Altitude>"
  Demux/3 -> Body Angles/3  "Yaw Angle"
  Demux/2 -> Body Angles/2  "Pitch Angle"
  Bus Selector/4 -> Heading/1  "<Heading>"
  Bus Selector/2 -> Demux1/1  "<V_b>"
  Bus Selector/1 -> Demux/1  "<phi_theta_psi>"
  Demux/1 -> Body Angles/1  "Roll Angle"
  Demux1/1 -> Body Velocities/1  "X Vel"
  Telemetry/1 -> Bus Selector/1

== system Copy_of_UAV/Flight Dynamics/Coeff Model/Actuator Aerodynamic Coefficients/Aileron ==
  Actuator : Inport
  Alpha : Inport  Port=2
  Constant1 : Constant  Value=0
  Constant2 : Constant  Value=0
  Constant3 : Constant  Value=0
  Constant4 : Constant  Value=aeroCoeff.Cy_da
  Constant5 : Constant  Value=aeroCoeff.Cl_da_alpha
  Constant6 : Constant  Value=aeroCoeff.Cn_da
  Constant7 : Constant  Value=aeroCoeff.Cl_da
  Mux1 : Mux  Inputs=6
  Product{1..5} (5 alike) : Product  SaturateOnIntegerOverflow=on  InputSameDT=on  OutDataTypeStr=Inherit: Same as first input
  Sum1 : Sum  Inputs=|++
  delCoeff : Outport
  wires:
  Product5/1 -> Sum1/2
  Constant7/1 -> Product5/1
  Sum1/1 -> Mux1/4
  Product4/1 -> Product1/1
  Alpha/1 -> Product4/1
  Constant6/1 -> Product3/2
  Product3/1 -> Mux1/6
  Actuator/1 -> Product2/1, Product3/1, Product5/2, Product4/2
  Product1/1 -> Sum1/1
  Constant5/1 -> Product1/2
  Constant4/1 -> Product2/2
  Constant3/1 -> Mux1/5
  Constant2/1 -> Mux1/3
  Constant1/1 -> Mux1/1
  Mux1/1 -> delCoeff/1
  Product2/1 -> Mux1/2

== system Copy_of_UAV/Flight Dynamics/Coeff Model/Actuator Aerodynamic Coefficients/Elevator ==
  Actuator : Inport
  Beta : Inport  Port=2
  Constant{1..2,4,8} (4 alike) : Constant  Value=0
  Constant5 : Constant  Value=aeroCoeff.Cz_de_beta
  Constant6 : Constant  Value=aeroCoeff.Cm_de
  Constant7 : Constant  Value=aeroCoeff.Cz_de
  Mux1 : Mux  Inputs=6
  Product1 : Product  SaturateOnIntegerOverflow=on  InputSameDT=on  OutDataTypeStr=Inherit: Same as first input
  Product2 : Product  SaturateOnIntegerOverflow=on  InputSameDT=on  OutDataTypeStr=Inherit: Same as first input
  Product3 : Product  SaturateOnIntegerOverflow=on  InputSameDT=on  OutDataTypeStr=Inherit: Same as first input
  Product4 : Product  Inputs=3  SaturateOnIntegerOverflow=on  InputSameDT=on  OutDataTypeStr=Inherit: Same as first input
  Sum : Sum  Inputs=|++
  delCoeff : Outport
  wires:
  Product2/1 -> Sum/2
  Beta/1 -> Product4/1, Product4/2
  Product3/1 -> Mux1/5
  Constant2/1 -> Mux1/6
  Constant8/1 -> Mux1/4
  Constant1/1 -> Mux1/1
  Product1/1 -> Sum/1
  Mux1/1 -> delCoeff/1
  Constant4/1 -> Mux1/2
  Constant7/1 -> Product2/1
  Product4/1 -> Product1/1
  Constant5/1 -> Product1/2
  Constant6/1 -> Product3/2
  Actuator/1 -> Product4/3, Product2/2, Product3/1
  Sum/1 -> Mux1/3

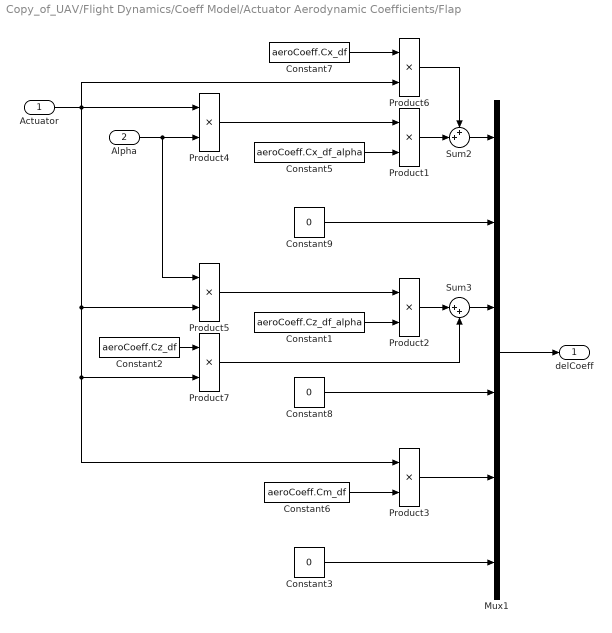
== system Copy_of_UAV/Flight Dynamics/Coeff Model/Actuator Aerodynamic Coefficients/Flap ==
  Actuator : Inport
  Alpha : Inport  Port=2
  Constant1 : Constant  Value=aeroCoeff.Cz_df_alpha
  Constant2 : Constant  Value=aeroCoeff.Cz_df
  Constant3 : Constant  Value=0
  Constant5 : Constant  Value=aeroCoeff.Cx_df_alpha
  Constant6 : Constant  Value=aeroCoeff.Cm_df
  Constant7 : Constant  Value=aeroCoeff.Cx_df
  Constant8 : Constant  Value=0
  Constant9 : Constant  Value=0
  Mux1 : Mux  Inputs=6
  Product{1..7} (7 alike) : Product  SaturateOnIntegerOverflow=on  InputSameDT=on  OutDataTypeStr=Inherit: Same as first input
  Sum2 : Sum  Inputs=++|
  Sum3 : Sum  Inputs=|++
  delCoeff : Outport
  wires:
  Product7/1 -> Sum3/2
  Product6/1 -> Sum2/1
  Product1/1 -> Sum2/2
  Constant1/1 -> Product2/2
  Product5/1 -> Product2/1
  Alpha/1 -> Product5/1, Product4/2
  Constant2/1 -> Product7/1
  Product2/1 -> Sum3/1
  Sum3/1 -> Mux1/3
  Sum2/1 -> Mux1/1
  Product3/1 -> Mux1/5
  Constant9/1 -> Mux1/2
  Constant8/1 -> Mux1/4
  Mux1/1 -> delCoeff/1
  Constant3/1 -> Mux1/6
  Constant7/1 -> Product6/1
  Product4/1 -> Product1/1
  Constant5/1 -> Product1/2
  Constant6/1 -> Product3/2
  Actuator/1 -> Product4/1, Product7/2, Product3/1, Product5/2, Product6/2

== system Copy_of_UAV/Flight Dynamics/Coeff Model/Actuator Aerodynamic Coefficients/Rudder ==
  Actuator : Inport
  Alpha : Inport  Port=2
  Constant1 : Constant  Value=aeroCoeff.Cx_dr
  Constant2 : Constant  Value=0
  Constant3 : Constant  Value=0
  Constant4 : Constant  Value=aeroCoeff.Cl_dr
  Constant5 : Constant  Value=aeroCoeff.Cy_dr_alpha
  Constant6 : Constant  Value=aeroCoeff.Cn_dr
  Constant7 : Constant  Value=aeroCoeff.Cy_dr
  Mux1 : Mux  Inputs=6
  Product{1..6} (6 alike) : Product  SaturateOnIntegerOverflow=on  InputSameDT=on  OutDataTypeStr=Inherit: Same as first input
  Sum1 : Sum  Inputs=|++
  delCoeff : Outport
  wires:
  Product6/1 -> Sum1/2
  Sum1/1 -> Mux1/2
  Product5/1 -> Mux1/1
  Constant1/1 -> Product5/2
  Product2/1 -> Mux1/4
  Product3/1 -> Mux1/6
  Constant4/1 -> Product2/2
  Product1/1 -> Sum1/1
  Mux1/1 -> delCoeff/1
  Constant3/1 -> Mux1/5
  Constant7/1 -> Product6/1
  Constant2/1 -> Mux1/3
  Alpha/1 -> Product4/1
  Product4/1 -> Product1/1
  Constant5/1 -> Product1/2
  Constant6/1 -> Product3/2
  Actuator/1 -> Product5/1, Product4/2, Product6/2, Product2/1, Product3/1
